simulink model "NonLinearModel"  (R2023b)
settings: Solver=ode45  StartTime=0.0  StopTime=Tsim*1.4  RelTol=1e-10  EnableMultiTasking=on
values from neighbouring files (symbols this model uses):
  alpha_init = 1*x_trim(1)    [FLYmodel.m]
  b = 9.17    [MyAircraft.mat]    (also in longMotion.m = 2.15; trimConfig.m)
  c = 2.15    [MyAircraft.mat]    (also in trimConfig.m)
  CG = 0.245    [MyAircraft.mat]    (also in trimConfig.m)
  el_init = x_trim(2)    [FLYmodel.m]
  eng_init = x_trim(4)    [FLYmodel.m]
  H_init = plane.h    [FLYmodel.m]
  Jgross = [5000 34000 45000 2200]    [MyAircraft.mat]    (also in trimConfig.m = [Ixx Iyy Izz Ixz])
  longK = lqr(podelny_system,Q,R)    [LQnavrh.m]
  m = 6500    [MyAircraft.mat]    (also in input_param.m = str2double(answerX{3}); trimConfig.m = plane.m)
  pitch_init = 1*x_trim(3)    [FLYmodel.m]
  plane = input_param    [FLYmodel.m]    (also in MyAircraft.mat = )
  rAC = 0.245    [MyAircraft.mat]    (also in trimConfig.m = plane.x_T)
  rho = 0.320310691736    [MyAircraft.mat]    (also in input_param.m = rho_0*(1-vyska/44308)^4.2553; trimConfig.m = plane.rho)
  S = 18.8    [MyAircraft.mat]    (also in latMotion.m; longMotion.m; trimConfig.m)
  Ts = 1/50    (= 0.02)    [FLYmodel.m]
  v0 = plane.v0    [FLYmodel.m]    (also in MyAircraft.mat = 187; input_param.m = str2double(answerX{1}); trimConfig.m)
  V_init = [plane.v0*cos(x_trim(1)) 0 plane.v0*sin(x_trim(1))]'    [FLYmodel.m]
  x_trim = trimConfig(plane)    [FLYmodel.m]    (also in MyAircraft.mat = [0.106204510792 -0.023384072427 0.106204510792 11783.3986038; trimConfig.m = [x(1) x(2) x(3) x(4)])
undefined symbols (not defined in the file or in its folder): Ap, As, Bp, Bs, Cp, Cs, Dp, Ds
libraries: simulink_extras x18
(part 1 of 2)
settings Model: Creator=Beruska  LastModifiedBy=cigla
settings SolverCC: ZeroCrossAlgorithm=Non-adaptive  AlgebraicLoopSolver=TrustRegion
settings DataIOCC: LimitDataPoints=on  SaveFormat=Array  SignalLoggingSaveFormat=ModelDataLogs  ReturnWorkspaceOutputs=off
settings OptimizationCC: ExpressionDepthLimit=2147483647  InitFltsAndDblsToZero=on  LifeSpan=inf
settings DebuggingCC: SaveWithDisabledLinksMsg=none  SaveWithParameterizedLinksMsg=none  UnderspecifiedInitializationDetection=Classic  MergeDetectMultiDrivingBlocksExec=none  SignalResolutionControl=TryResolveAllWithWarning  MultiTaskDSMMsg=warning  MultiTaskCondExecSysMsg=none  FcnCallInpInsideContextMsg=warning  StateNameClashWarn=warning  SFUnexpectedBacktrackingDiag=warning  SFNoUnconditionalDefaultTransitionDiag=warning  SFExecutionAtInitializationDiag=none  ArithmeticOperatorsInVariantConditions=warning
settings HardwareCC: ProdBitPerPointer=32  ProdBitPerSizeT=32  ProdBitPerPtrDiffT=32  ProdLargestAtomicFloat=None  ProdIntDivRoundTo=Undefined  ProdEndianess=Unspecified  ProdWordSize=32  ProdHWDeviceType=32-bit Generic  TargetHWDeviceType=32-bit Generic
settings ModelReferenceCC: PropagateSignalLabelsOutOfModel=off
settings SFSimCC: SimParseCustomCode=off
settings CodeAppCC: StateflowObjectComments=on
settings GRTTargetCC: TargetFcnLib=ansi_tfl_tmw.mat  TargetLangStandard=C89/C90 (ANSI)  CombineOutputUpdateFcns=off  GRTInterface=on
settings ConfigComp: CovMetricSettings=dw  CovSaveCumulativeToWorkspaceVar=on  CovSaveSingleToWorkspaceVar=on

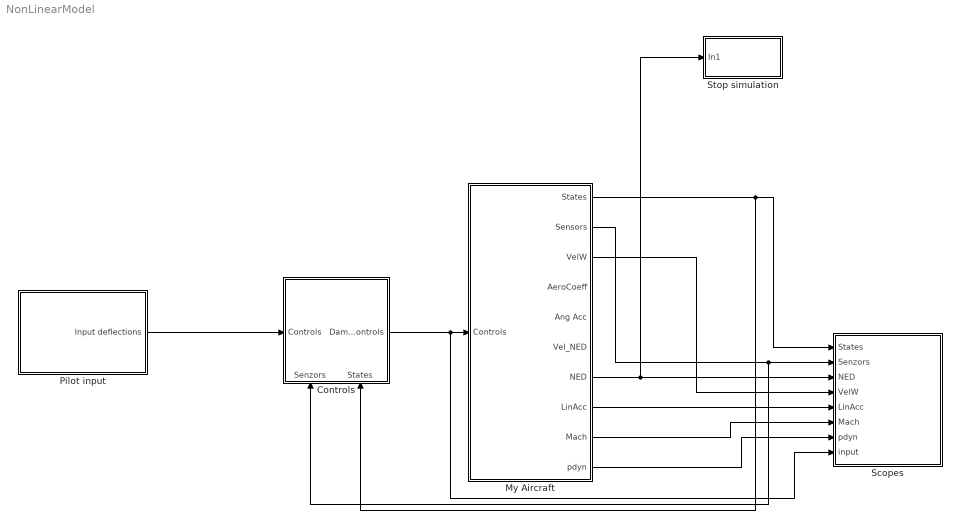
== system NonLinearModel ==
  Controls : Subsystem
      settings: PortSchema="{\"entries\":[{\"content\":{\"sides\":[{\"content\":{\"connectorIds\":[\"In1\"]},\"type\":\"ConnectorPlacement.EquallySpacedRectSide\",\"uuid\":\"4b7104ba-33e9-4b34-bfe8-b4b6035b4af3\"},{\"content\":{\"connectorIds\":[\"Out1\"],\"side\":\"RIGHT\"},\"type\":\"ConnectorPlacement.EquallySpacedRectSide\",\"uuid\":\"7145cc92-5786-41d0-90fc-f90dc0f3b476\"},{\"content\":{\"side\":\"TOP\"},\"type\":\"ConnectorPlacement.EquallySpacedRectSide\",\"uuid\":\"eba59bfa-479c-4b8a-8384-c15642ccc9eb\"},{\"content\":{\"connectorIds\":[\"In2\",\"In3\"],\"side\":\"BOTTOM\"},\"type\":\"ConnectorPlacement.EquallySpacedRectSide\",\"uuid\":\"538b7866-be33-4433-b066-8ee0a3ce190d\"}]},\"type\":\"ConnectorPlacement.EquallySpacedConnector\",\"uuid\":\"caacbf69-b2ca-40be-96e6-630faa4c76a7\"}],\"packageUris\":[\"http://schema.mathworks.com/mf0/Connector/R2020b\"],\"version\":\"1.0\"}"
  My Aircraft : Subsystem  mask(6-DOF Aircraft Model){aircraftcfg='MyAircraft.mat', VelocitiesIni=V_init, RatesIni=[0 0 0]', EulerIni=[0 pitch_init 0], PositionIni=[45/180*pi 45/180*pi H_init], QuatIni=[1 0 0 0], tsamp=Ts}
      mask prompts: aircraftcfg "Aircraft configuration file:"; VelocitiesIni "Initial velocities:"; RatesIni "Initial angular rates:"; EulerIni "Initial Euler:"; PositionIni "Initial position:"; QuatIni "Initial attitude:"; tsamp "Sample time:"
      mask help: Nonlinear 6-DOF aircraft model with equations of motion in body frame.
      mask init:
      | load(aircraftcfg);
      mask Help:
      | The block implements the 6-DOF nonlinear aircraft model using AeroSim blocks. Velocities are computed in body frame.
      | <P><B>Inputs:</B>
      | <LI>Controls = the 7x1 vector of aircraft controls [flap elevator aileron rudder throttle mixture ignition]. Aerodynamic controls are in radians, throttle is from 0 to 1, mixture is fraction air/fuel flow, ignition is 0 (engine off) or 1 (engine on).</LI>
      | <LI>Winds = the 3x1 vector of background wind speed components in navigation frame [North East Down]</LI>
      | <LI>RST = the integrator reset flag (0 or 1, all integrators on rising edge)
      | </P>
      | <P><B>Outputs:</B>
      | <LI>States = the 15x1 aircraft state vector [Velocities, Angular rates, Quaternions, Position, Fuel mass, Engine speed].</LI>
      | <LI>Sensors = the 18x1 vector of sensor outputs [GPS Position, GPS Groundspeed, Accelerometers, Gyros, Air data, Magnetometer].</LI>
      | <LI>VelW = the 3x1 vector of aircraft velocity in wind axes [Airspeed, sideslip, angle of attack]</LI>
      | <LI>Mach = the Mach number</LI>
      | <LI>Ang Acc = the 3x1 vector of angular accelerations
      | <LI>Euler = the 3x1 vector of Euler angles (roll, pitch, yaw)</LI>
      | <LI>AeroCoeff = the 6x1 vector of aerodynamic coefficients [CD CY CL Cl Cm Cn]</LI>
      | <LI>PropCoeff = the 3x1 vector of propeller coefficients [J CT CP]</LI>
      | <LI>EngCoeff = the 5x1 vector of engine coefficients [MAP Airflow Fuelflow BSFC Power]</LI>
      | <LI>Mass = the current aircraft mass</LI>
      | <LI>ECEF = 3x1 vector of position of the aircraft in the Earth-centered, Earth-fixed frame</LI>
      | <LI>MSL = the aircraft altitude above mean-sea-level</LI>
      | <LI>AGL = the aircraft altitude above terrain</LI>
      | <LI>REarth = the Earth equivalent radius at current location
      | <LI>AConGnd = the aircraft-on-ground flag (0 if aircraft above ground, 1 if aircraft on the ground)</LI>
      | </P>
      | <P><B>Parameters:</B>
      | <LI>Aircraft configuration file = the MAT-file with aircraft data</LI>
      | <LI>Initial velocities = the 3x1 vector of initial aircraft velocities in body axes [u v w]</LI>
      | <LI>Initial angular rates = the 3x1 vector of initial angular rates [p q r]</LI>
      | <LI>Initial attitude = the 4x1 vector of initial quaternions [e0 ex ey ez]</LI>
      | <LI>Initial position = the 3x1 vector of initial aircraft location [Lat Lon Alt]</LI>
      | <LI>Initial fuel mass = the initial quantity of fuel on-board the aircraft</LI>
      | <LI>Initial engine speed = the initial engine rotation speed</LI>
      | <LI>Ground altitude = the ground altitude at aircraft location</LI>
      | <LI>WMM coefficient file = the path to the magnetic model coefficient file</LI>
      | <LI>Simulation date = the date to be used for the magnetic model [day month year]</LI>
      | <LI>Sample time = the aircraft model sample time.</LI>
      | </P>
  Pilot input : Subsystem
  Scopes : Subsystem
  Stop simulation : Subsystem
  wires:
  My Aircraft/3(VelW) -> Scopes/4(VelW)
  My Aircraft/2(Sensors) -> Scopes/2(Senzors), Controls/2(Senzors)
  My Aircraft/7(NED) -> Stop simulation/1(In1), Scopes/3(NED)
  My Aircraft/1(States) -> Scopes/1(States), Controls/3(States)
  My Aircraft/8(LinAcc) -> Scopes/5(LinAcc)
  My Aircraft/9("Mach ") -> Scopes/6(Mach)
  My Aircraft/10(pdyn) -> Scopes/7(pdyn)
  Pilot input/1(Input deflections) -> Controls/1(Controls)
  Controls/1(Damped controls) -> Scopes/8(input), My Aircraft/1(Controls)

== system NonLinearModel/Controls ==
  Controls : Inport
  Senzors : Inport  Port=2
  States : Inport  Port=3
  Add1 : Sum
  Damping of controls : Subsystem
  Delay : Delay  DelayLength=10
  Knob : KnobBlock  ScaleMin=-90  ScaleMax=90
  Knob1 : KnobBlock  ScaleMin=-90  ScaleMax=90
  Manual Switch : ManualSwitch
  Subsystem : Subsystem
  Subsystem1 : Subsystem
  pitch : Constant  Value=8.570086669921878
  roll : Constant  Value=0  OutDataTypeStr=Inherit: Inherit via back propagation
  Damped controls : Outport
  wires:
  Senzors/1 -> Subsystem1/1(In1), Damping of controls/2(Senzors), Subsystem/3(sensors)
  Controls/1 -> Add1/1
  Damping of controls/1(Damped controls) -> Damped controls/1  "Damped controls"
  Add1/1 -> Damping of controls/1(Controls from pilot)
  roll/1 -> Delay/1  "roll"
  pitch/1 -> Subsystem/2(pitch setpoint)
  Manual Switch/1 -> Add1/2
  Delay/1 -> Subsystem/1(roll stepoint)
  States/1 -> Subsystem/4(States)
  Subsystem/1(Out1) -> Manual Switch/1

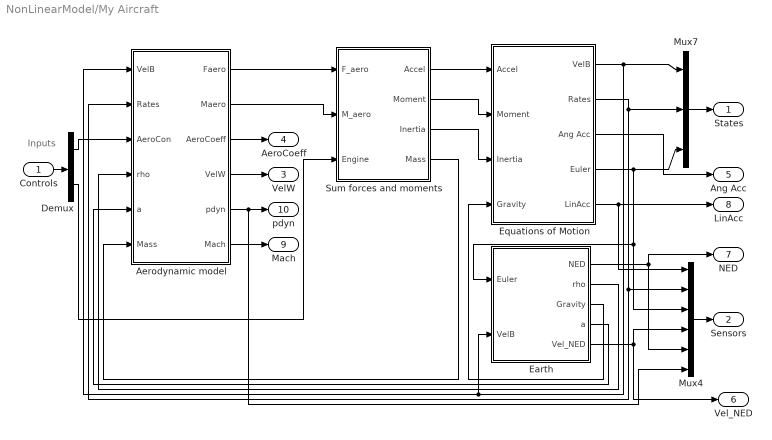
== system NonLinearModel/My Aircraft ==
  note: Inputs
  Controls : Inport
  Aerodynamic model : Subsystem
  Demux : Demux  Outputs=[3 1]
      settings: DisplayOption=none
  Earth : Subsystem
  Equations of Motion : Subsystem
  Mux4 : Mux  Inputs=6
  Mux7 : Mux  Inputs=3
  Sum forces and moments : Subsystem
  States : Outport
  Sensors : Outport  Port=2
  VelW : Outport  Port=3
  AeroCoeff : Outport  Port=4
  Ang Acc : Outport  Port=5
  Vel_NED : Outport  Port=6
  NED : Outport  Port=7
  LinAcc : Outport  Port=8
  "Mach " : Outport  Port=9
  pdyn : Outport  Port=10
  wires:
  Controls/1 -> Demux/1
  Mux4/1 -> Sensors/1
  Mux7/1 -> States/1
  Equations of Motion/1(VelB) -> Mux7/1, Aerodynamic model/1(VelB), Earth/2(VelB)
  Equations of Motion/2(Rates) -> Aerodynamic model/2(Rates), Mux4/2, Mux7/2
  Aerodynamic model/3(AeroCoeff) -> AeroCoeff/1
  Demux/1 -> Aerodynamic model/3(AeroCon)
  Earth/3(Gravity) -> Equations of Motion/4(Gravity)
  Equations of Motion/4(Euler) -> Mux7/3, Mux4/3, Earth/1(Euler)
  Aerodynamic model/1(Faero) -> Sum forces and moments/1(F_aero)
  Aerodynamic model/2(Maero) -> Sum forces and moments/2(M_aero)
  Demux/2 -> Sum forces and moments/3(Engine)
  Sum forces and moments/1(Accel) -> Equations of Motion/1(Accel)
  Sum forces and moments/2(Moment) -> Equations of Motion/2(Moment)
  Sum forces and moments/3(Inertia) -> Equations of Motion/3(Inertia)
  Earth/4(a) -> Aerodynamic model/5(a)
  Earth/2(rho) -> Aerodynamic model/4(rho)
  Earth/1(NED) -> Mux4/5, NED/1
  Aerodynamic model/5(pdyn) -> Mux4/6, pdyn/1
  Sum forces and moments/4(Mass) -> Aerodynamic model/6(Mass)
  Equations of Motion/3(Ang Acc) -> Ang Acc/1
  Equations of Motion/5(LinAcc) -> LinAcc/1, Mux4/1
  Aerodynamic model/6("Mach ") -> "Mach "/1
  Earth/5(Vel_NED) -> Vel_NED/1, Mux4/4
  Aerodynamic model/4(VelW) -> VelW/1

== system NonLinearModel/Pilot input ==
  Ground : Ground
  Ground1 : Ground
  Ground2 : Ground
  Manual Switch : ManualSwitch  CurrentSetting=0
  Manual Switch1 : ManualSwitch  CurrentSetting=0
  Manual Switch2 : ManualSwitch
  Mux3 : Mux
  Sum2 : Sum  Inputs=++|
  aileron : Subsystem
  elevator : Constant  Value=el_init
  elvator : Subsystem
  engine : Constant  Value=eng_init
  rudder : Subsystem
  Input deflections : Outport
  wires:
  engine/1 -> Mux3/4
  elevator/1 -> Sum2/2
  Sum2/1 -> Mux3/1
  Manual Switch/1 -> Mux3/2
  Ground/1 -> Manual Switch/2
  rudder/1(Out1) -> Manual Switch1/1  "rudder"
  Ground1/1 -> Manual Switch1/2
  Manual Switch1/1 -> Mux3/3
  elvator/1(Out1) -> Manual Switch2/1
  aileron/1(Out1) -> Manual Switch/1  "aileron"
  Ground2/1 -> Manual Switch2/2
  Manual Switch2/1 -> Sum2/1
  Mux3/1 -> Input deflections/1

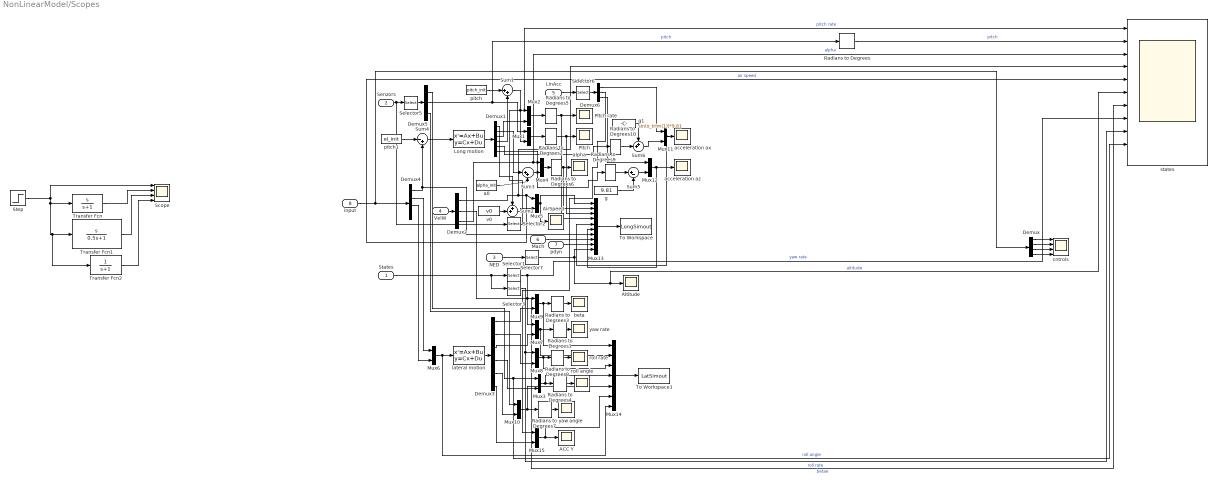
== system NonLinearModel/Scopes ==
  States : Inport
  Senzors : Inport  Port=2
  NED : Inport  Port=3
  VelW : Inport  Port=4
  LinAcc : Inport  Port=5
  Mach : Inport  Port=6
  pdyn : Inport  Port=7
  input : Inport  Port=8
  ACC Y : Scope
  AirSpeed : Scope
  Altitude : Scope
  Demux : Demux
  Demux1 : Demux  Outputs=6
      settings: DisplayOption=none
  Demux2 : Demux  Outputs=3
      settings: DisplayOption=none
  Demux3 : Demux  Outputs=6
      settings: DisplayOption=none
  Demux4 : Demux
      settings: DisplayOption=none
  Demux5 : Demux  Outputs=3
      settings: DisplayOption=none
  Demux6 : Demux  Outputs=3
      settings: DisplayOption=none
  Long motion : StateSpace  A=Ap  B=Bp  C=Cp  D=Dp  InitialCondition=0
  Mux{1..12,15} (13 alike) : Mux  Inputs=2
  Mux13 : Mux  Inputs=10
  Mux14 : Mux  Inputs=7
  Pitch : Scope
  Pitch rate : Scope
  Radians to Degrees{,1..8} (9 alike) : simulink_extras/Transformations/Radians to Degrees
  Radians to Degrees10 : simulink_extras/Transformations/Radians to Degrees
      link override Gain: Gain=9.81
  Radians to Degrees9 : simulink_extras/Transformations/Radians to Degrees
      link override Gain: Gain=-9.81
  Scope : Scope  NumInputPorts=4
  Selector1 : Selector  InputPortWidth=9  IndexOptions=Index vector (dialog)  Indices=6  OutputSizes=[(-2)]
  Selector2 : Selector  InputPortWidth=16  IndexOptions=Index vector (dialog)  Indices=5  OutputSizes=[(-2)]
  Selector3 : Selector  InputPortWidth=9  IndexOptions=Index vector (dialog)  Indices=4  OutputSizes=[(-2)]
  Selector5 : Selector  InputPortWidth=16  IndexOptions=Index vector (dialog)  Indices=[7 8 9]  OutputSizes=1
  Selector6 : Selector  InputPortWidth=3  IndexOptions=Index vector (dialog)  Indices=[1 2 3]  OutputSizes=1
  Selector7 : Selector  InputPortWidth=3  IndexOptions=Index vector (dialog)  Indices=3  OutputSizes=[(-2)]
  Step : Step  SampleTime=0
  Sum1 : Sum  Inputs=|++
  Sum2 : Sum  Inputs=++|
  Sum3 : Sum  Inputs=|++
  Sum4 : Sum  Inputs=|-+
  Sum5 : Sum  Inputs=|+-
  Sum6 : Sum  Inputs=++|
  To Workspace : ToWorkspace  VariableName=LongSimout  SaveFormat=Structure With Time  SampleTime=Ts
  To Workspace1 : ToWorkspace  VariableName=LatSimout  SaveFormat=Structure With Time  SampleTime=Ts
  Transfer Fcn : TransferFcn  Numerator=[1 0]  Denominator=[1 1]
  Transfer Fcn1 : TransferFcn  Numerator=[1 0]  Denominator=[0.5 1]
  Transfer Fcn2 : TransferFcn  Denominator=[1 1]
  a0 : Constant  Value=alpha_init
  acceleration ax : Scope
  acceleration az : Scope
  "alpha " : Scope
  beta : Scope
  cntrols : Scope  NumInputPorts=4
  g : Constant  Value=9.81
  g1 : Constant  Value=sin(x_trim(1))*9.81
  lateral motion : StateSpace  A=As  B=Bs  C=Cs  D=Ds  InitialCondition=0
  pitch : Constant  Value=pitch_init
  pitch1 : Constant  Value=el_init
  roll angle : Scope
  roll rate : Scope
  states : Scope  NumInputPorts=11
  v0 : Constant  Value=v0
  yaw angle : Scope
  yaw rate : Scope
  wires:
  Long motion/1 -> Demux1/1
  Demux1/4 -> Sum1/2
  Mux1/1 -> Radians to Degrees2/1
  pitch/1 -> Sum1/1
  Demux5/2 -> Radians to Degrees/1, Mux1/1  "pitch"
  Mux2/1 -> Radians to Degrees5/1
  Demux1/3 -> Mux2/2
  Mux4/1 -> Radians to Degrees6/1
  Demux1/2 -> Sum3/1
  Demux1/1 -> Sum2/1
  Mux5/1 -> AirSpeed/1, Mux13/1
  Sum2/1 -> Mux5/2
  v0/1 -> Sum2/2
  Sum3/1 -> Mux4/2
  a0/1 -> Sum3/2
  Selector1/1 -> Mux7/1, states/8  "yaw rate"
  Mux7/1 -> Mux14/2, Radians to Degrees1/1
  Radians to Degrees1/1 -> yaw rate/1
  Mux8/1 -> Radians to Degrees8/1, Mux14/3
  Radians to Degrees8/1 -> roll rate/1
  Selector3/1 -> Mux8/1, states/9  "roll rate"
  lateral motion/1 -> Demux3/1
  Mux9/1 -> Radians to Degrees3/1, Mux14/1
  Radians to Degrees3/1 -> beta/1
  Mux6/1 -> lateral motion/1, Mux14/7
  Demux4/3 -> Mux6/2
  Demux4/1 -> Sum4/2, Mux13/7
  Demux2/3 -> states/3, Mux4/1  "alpha"
  input/1 -> Demux/1, Demux4/1
  Demux4/2 -> Mux6/1
  Sum4/1 -> Long motion/1
  pitch1/1 -> Sum4/1
  Demux3/2 -> Mux8/2
  Demux3/1 -> Mux9/2
  VelW/1 -> Demux2/1
  Demux2/2 -> states/7, Mux9/1  "betae"
  Radians to Degrees6/1 -> "alpha "/1, Mux13/2
  Selector2/1 -> states/1, Mux2/1  "pitch rate"
  Radians to Degrees5/1 -> Pitch rate/1, Mux13/4
  Demux3/3 -> Mux7/2
  Mux3/1 -> Radians to Degrees4/1, Mux14/4
  Radians to Degrees4/1 -> roll angle/1
  Demux3/4 -> Mux3/2
  Senzors/1 -> Selector2/1, Selector5/1
  Demux5/3 -> Mux10/1
  Mux10/1 -> Radians to Degrees7/1, Mux14/5
  Radians to Degrees7/1 -> yaw angle/1
  Demux3/5 -> Mux10/2
  Demux5/1 -> Mux3/1, states/10  "roll angle"
  Selector5/1 -> Demux5/1
  Radians to Degrees2/1 -> Pitch/1, Mux13/3
  Sum1/1 -> Mux1/2
  States/1 -> Selector1/1, Selector3/1
  Demux2/1 -> states/5, Mux5/1, states/4  "air speed"
  Demux1/5 -> Radians to Degrees10/1
  Mux11/1 -> acceleration ax/1, Mux13/5
  Selector6/1 -> Demux6/1
  Demux6/1 -> Mux11/1
  Mux12/1 -> Mux13/6, acceleration az/1
  Demux6/3 -> Mux12/1
  Demux1/6 -> Radians to Degrees9/1
  Radians to Degrees9/1 -> Sum5/1
  LinAcc/1 -> Selector6/1
  g/1 -> Sum5/2
  Sum5/1 -> Mux12/2
  g1/1 -> Sum6/1
  Radians to Degrees10/1 -> Sum6/2
  Sum6/1 -> Mux11/2
  Mux13/1 -> To Workspace/1
  Mach/1 -> Mux13/8
  pdyn/1 -> Mux13/9
  NED/1 -> Selector7/1
  Selector7/1 -> Mux13/10, states/6, Altitude/1  "altitude"
  Mux14/1 -> To Workspace1/1
  Demux6/2 -> Mux15/1
  Mux15/1 -> ACC Y/1, Mux14/6
  Demux3/6 -> Mux15/2
  Transfer Fcn/1 -> Scope/2
  Step/1 -> Transfer Fcn/1, Transfer Fcn2/1, Transfer Fcn1/1, Scope/1
  Transfer Fcn1/1 -> Scope/3
  Transfer Fcn2/1 -> Scope/4
  Demux/1 -> cntrols/1
  Demux/2 -> cntrols/2
  Demux/3 -> cntrols/3
  Demux/4 -> cntrols/4
  Radians to Degrees/1 -> states/2  "pitch"

== system NonLinearModel/Stop simulation ==
  In1 : Inport
  Constant : Constant  Value=0
  Constant1 : Constant
  Demux : Demux  Outputs=[2 1]
  Scope1 : Scope
  Stop Simulation : Stop
  Switch : Switch  SaturateOnIntegerOverflow=off  InputSameDT=off
  Terminator : Terminator
  wires:
  Constant/1 -> Switch/1
  Constant1/1 -> Switch/3
  In1/1 -> Demux/1
  Demux/2 -> Switch/2
  Demux/1 -> Terminator/1
  Switch/1 -> Stop Simulation/1, Scope1/1

== system NonLinearModel/Controls/Damping of controls ==
  Controls from pilot : Inport
  Senzors : Inport  Port=2
  Add{,2..3,5} (4 alike) : Sum
  Demux1 : Demux  Outputs=3
  Demux2 : Demux
  Gain2 : Gain  Gain=0.07
  Ground : Ground
  Mux : Mux
  Subsystem : Subsystem
  Transfer Fcn : TransferFcn  Numerator=[1 0]  Denominator=[1 1]
  pitch damper : Gain  Gain=0.063
  roll damper : Gain  Gain=-0.054
  Damped controls : Outport
  wires:
  pitch damper/1 -> Add/2
  Add/1 -> Mux/1  "damped elevator"
  Demux2/1 -> Add/1  "elevator from pilot"
  Demux1/3 -> roll damper/1  "roll rate"
  Demux2/4 -> Add3/1  "Engine thrust from pilot"
  Demux2/3 -> Add5/1  "Rudder from pilot"
  Demux1/2 -> pitch damper/1  "pitch rate"
  Demux1/1 -> Gain2/1  "yaw rate"
  Add3/1 -> Mux/4  "engine"
  Add5/1 -> Mux/3  "damped rudder"
  Demux2/2 -> Add2/1  "Aileron from pilot"
  Add2/1 -> Mux/2  "damped ailerons"
  Controls from pilot/1 -> Demux2/1
  Mux/1 -> Damped controls/1
  roll damper/1 -> Add2/2
  Transfer Fcn/1 -> Add5/2
  Gain2/1 -> Transfer Fcn/1
  Ground/1 -> Add3/2
  Senzors/1 -> Subsystem/1(In1)
  Subsystem/1(Rates) -> Demux1/1

== system NonLinearModel/Controls/Subsystem ==
  roll stepoint : Inport
  pitch setpoint : Inport  Port=2
  sensors : Inport  Port=3
  States : Inport  Port=4
  Constant : Constant  Value=0
  Manual Switch : ManualSwitch  CurrentSetting=0
  Mux : Mux
  PAH : Subsystem
  PAH_LQ : Subsystem
  RAH : Subsystem
  RAH_LQ : Subsystem
  demuxing hell : Subsystem
  Out1 : Outport
  wires:
  Mux/1 -> Out1/1
  roll stepoint/1 -> RAH/1(In1)
  RAH/1(Out1) -> Mux/2  "aileron"
  pitch setpoint/1 -> PAH_LQ/1(pitch setpoint), PAH/1(pitch setpoint)
  Manual Switch/1 -> Mux/1  "elevator"
  ? -> Mux/3  "rudder"
  ? -> Mux/4  "engine"
  sensors/1 -> demuxing hell/1(sensors)
  States/1 -> demuxing hell/2(In2)
  demuxing hell/1(pitch) -> PAH/2(pitch)
  demuxing hell/2(roll) -> RAH/2(roll)
  demuxing hell/3(long states) -> PAH_LQ/2(long states)
  PAH/1(Out1) -> Manual Switch/1  "elevator"
  PAH_LQ/1(Out1) -> Manual Switch/2

== system NonLinearModel/Controls/Subsystem1 ==
  In1 : Inport
  Demux : Demux  Outputs=6
  Terminator{,1..5} (6 alike) : Terminator
  wires:
  Demux/1 -> Terminator/1  "Lin Acc"
  Demux/2 -> Terminator1/1  "Rates"
  Demux/3 -> Terminator5/1  "Euler Angles"
  Demux/5 -> Terminator3/1  "NED"
  Demux/4 -> Terminator2/1  "Velocity NED"
  Demux/6 -> Terminator4/1  "dynamic pressure"
  In1/1 -> Demux/1

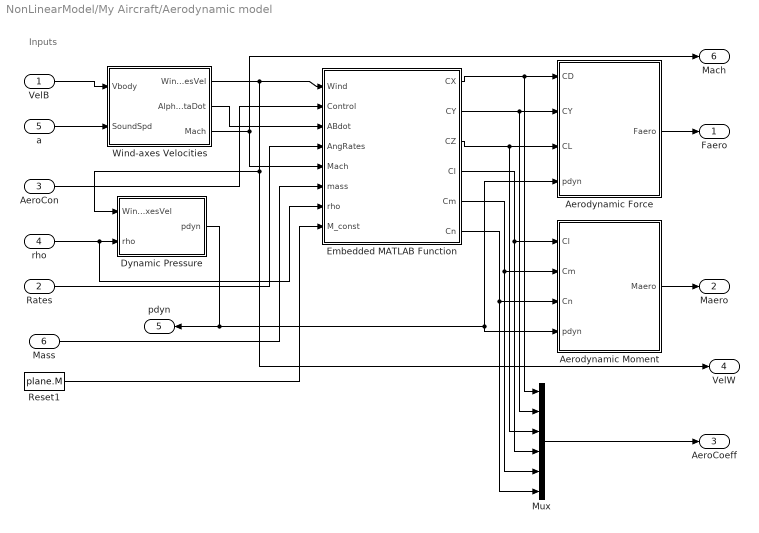
== system NonLinearModel/My Aircraft/Aerodynamic model ==
  note: Inputs
  VelB : Inport  PortDimensions=[3 1]
  Rates : Inport  Port=2  PortDimensions=[3 1]
  AeroCon : Inport  Port=3
  rho : Inport  Port=4  PortDimensions=1
  a : Inport  Port=5  PortDimensions=1
  Mass : Inport  Port=6
  Aerodynamic Force : Subsystem  mask(Aerodynamic force){S=S}
      mask prompts: S "Wing reference area:"
      mask help: Computes aerodynamic force in body axes.
      mask Help:
      | The block computes the aerodynamic force in body axes.
      | <P><B>Inputs:</B>
      | <LI>CD = the coefficient of drag</LI>
      | <LI>CY = the coefficient of side force</LI>
      | <LI>CL = the coefficient of lift</LI>
      | <LI>pdyn = the dynamic pressure</LI>
      | <LI>WindAxesVel = the 3x1 vector of wind axes velocity components [Va beta alpha]'</LI>
      | </P>
      | <P><B>Output:</B> the 3x1 vector of aerodynamic forces in body axes</P>
      | <P><B>Parameters:</B>
      | <LI>S = the wing reference area</LI>
      | </P>
  Aerodynamic Moment : Subsystem  mask(Aerodynamic moment){c=c, b=b, S=S}
      mask prompts: c "Mean aerodynamic chord:"; b "Wing span:"; S "Wing reference area:"
      mask help: Computes aerodynamic moment with respect to the aerodynamic center.
  Dynamic Pressure : Subsystem
  Embedded MATLAB Function : MATLAB Function  TreatAsAtomicUnit=on
  Mux : Mux  Inputs=6
  Reset1 : Constant  Value=plane.M
  Wind-axes Velocities : Subsystem
  Faero : Outport
  Maero : Outport  Port=2
  AeroCoeff : Outport  Port=3
  VelW : Outport  Port=4
  pdyn : Outport  Port=5
  "Mach " : Outport  Port=6
  wires:
  Rates/1 -> Embedded MATLAB Function/4(AngRates)
  Aerodynamic Moment/1(Maero) -> Maero/1
  Aerodynamic Force/1(Faero) -> Faero/1
  Dynamic Pressure/1(pdyn) -> Aerodynamic Moment/4(pdyn), Aerodynamic Force/4(pdyn), pdyn/1
  Wind-axes Velocities/2(AlphaBetaDot) -> Embedded MATLAB Function/3(ABdot)
  rho/1 -> Dynamic Pressure/2(rho), Embedded MATLAB Function/7(rho)
  Wind-axes Velocities/1(WindAxesVel) -> Dynamic Pressure/1(WindAxesVel), VelW/1, Embedded MATLAB Function/1(Wind)
  a/1 -> Wind-axes Velocities/2(SoundSpd)
  VelB/1 -> Wind-axes Velocities/1(Vbody)
  Wind-axes Velocities/3(Mach) -> "Mach "/1, Embedded MATLAB Function/5(Mach)
  AeroCon/1 -> Embedded MATLAB Function/2(Control)
  Embedded MATLAB Function/1(CX) -> Aerodynamic Force/1(CD), Mux/1
  Embedded MATLAB Function/3(CZ) -> Aerodynamic Force/3(CL), Mux/3
  Embedded MATLAB Function/5(Cm) -> Aerodynamic Moment/2(Cm), Mux/5
  Embedded MATLAB Function/2(CY) -> Aerodynamic Force/2(CY), Mux/2
  Embedded MATLAB Function/6(Cn) -> Aerodynamic Moment/3(Cn), Mux/6
  Reset1/1 -> Embedded MATLAB Function/8(M_const)
  Embedded MATLAB Function/4(Cl) -> Aerodynamic Moment/1(Cl), Mux/4
  Mass/1 -> Embedded MATLAB Function/6(mass)
  Mux/1 -> AeroCoeff/1

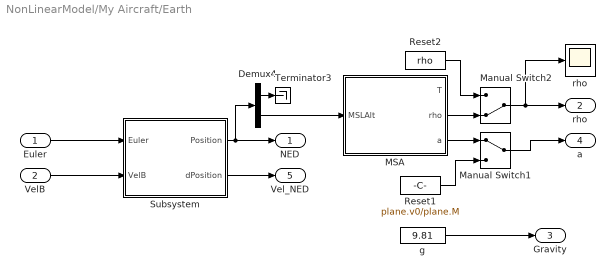
== system NonLinearModel/My Aircraft/Earth ==
  Euler : Inport  OutDataTypeStr=double
  VelB : Inport  Port=2  OutDataTypeStr=double
  Demux4 : Demux  Outputs=[2 1]
      settings: DisplayOption=none
  MSA : Subsystem
  Manual Switch1 : ManualSwitch
  Manual Switch2 : ManualSwitch  CurrentSetting=0
  Reset1 : Constant  Value=plane.v0/plane.M
  Reset2 : Constant  Value=rho
  Subsystem : Subsystem
  Terminator3 : Terminator
  g : Constant  Value=9.81
  "rho " : Scope
  NED : Outport
  rho : Outport  Port=2
  Gravity : Outport  Port=3
  a : Outport  Port=4
  Vel_NED : Outport  Port=5
  wires:
  g/1 -> Gravity/1
  MSA/3(a) -> Manual Switch1/1
  Manual Switch1/1 -> a/1
  MSA/2(rho) -> Manual Switch2/2
  Reset2/1 -> Manual Switch2/1
  Manual Switch2/1 -> rho/1, "rho "/1
  Demux4/1 -> Terminator3/1
  Subsystem/1(Position) -> Demux4/1, NED/1
  Reset1/1 -> Manual Switch1/2
  Euler/1 -> Subsystem/1(Euler)
  VelB/1 -> Subsystem/2(VelB)
  Demux4/2 -> MSA/1(MSLAlt)
  Subsystem/2(dPosition) -> Vel_NED/1

== system NonLinearModel/My Aircraft/Equations of Motion ==
  note: Inputs
  note: Outputs
  Accel : Inport  PortDimensions=[3 1]
  Moment : Inport  Port=2  PortDimensions=[3 1]
  Inertia : Inport  Port=3  PortDimensions=[4 1]
  Gravity : Inport  Port=4
  Forces : Subsystem  mask(Force equations){VelocitiesIni=VelocitiesIni}
      mask prompts: VelocitiesIni "Initial velocities:"
      mask help: 6-DOF rigid body force equations.
      mask Help:
      | The block implements the 6-DOF rigid-body force equations.
      | <P><B>Inputs:</B>
      | <LI>Rates = the 3x1 vector of body angular rates</LI>
      | <LI>Accel = the 3x1 vector of linear body accelerations</LI>
      | <LI>Gravity = the gravitational acceleration at current location.
      | <LI>DCM = the 3x3 rotation matrix from navigation to body frame.
      | <LI>RST = the integrator reset flag (rising edge)</LI>
      | </P>
      | <P><B>Output:</B>
      | <LI>Velocities = the 3x1 vector of aircraft velocities in body axes</LI>
      | </P>
      | <P><B>Parameters:</B>
      | <LI>Initial velocities = the 3x1 vector of initial aircraft velocities</LI>
      | </P>
  Kinematics (Euler) : Subsystem  mask(Kinematic Equations){EulerIniX=EulerIni}
      mask prompts: EulerIniX "Initial Euler:"
      mask help: 6-DOF rigid body kinematic equations, using Euler-Rodrigues quaternions.
      mask Help:
      | The block implements the 6-DOF rigid-body kinematic equations, using Euler-Rodrigues quaternions.
      | <P><B>Inputs:</B>
      | <LI>Rates = the 3x1 vector of body angular rates</LI>
      | <LI>RST = the integrator reset flag (rising edge)</LI>
      | </P>
      | <P><B>Output:</B>
      | <LI>Quaternions = the 4x1 vector of body quaternions</LI>
      | </P>
      | <P><B>Parameters:</B>
      | <LI>Initial quaternions = the 4x1 vector of initial body quaternions</LI>
      | </P>
  Moments : Subsystem  mask(Moment equations){RatesIni=RatesIni}
      mask prompts: RatesIni "Initial angular rates:"
      mask help: 6-DOF rigid body moment equations.
      mask Help:
      | The block implements the 6-DOF rigid-body moment equations.
      | <P><B>Inputs:</B>
      | <LI>Inertia = the 10x1 vector of inertia coefficients</LI>
      | <LI>Moments = the 3x1 vector of airframe moments</LI>
      | <LI>RST = the integrator reset flag (rising edge)</LI>
      | </P>
      | <P><B>Output:</B>
      | <LI>Angular Rates = the 3x1 vector of body angular rates</LI>
      | <LI>Angular Acc = the 3x1 vector of body angular accelerations.
      | </P>
      | <P><B>Parameters:</B>
      | <LI>Initial rates = the 3x1 vector of initial angular rates</LI>
      | </P>
  VelB : Outport
  Rates : Outport  Port=2
  Ang Acc : Outport  Port=3
  Euler : Outport  Port=4
  LinAcc : Outport  Port=5
  wires:
  Moments/2(Angular Acc) -> Ang Acc/1
  Moments/1(Angular Rates) -> Rates/1, Kinematics (Euler)/1(Rates), Forces/1(Rates)
  Forces/1(Velocities) -> VelB/1
  Inertia/1 -> Moments/1(Inertia)
  Moment/1 -> Moments/2(Moments)
  Accel/1 -> Forces/2(Accel)
  Kinematics (Euler)/1(Euler) -> Forces/3(Euler), Euler/1
  Gravity/1 -> Forces/4(Gravity)
  Forces/2(LinAcc) -> LinAcc/1

== system NonLinearModel/My Aircraft/Sum forces and moments ==
  F_aero : Inport
  M_aero : Inport  Port=2
  Engine : Inport  Port=3
  CG location : Constant  Value=CG
  Mass gross : Constant  Value=m
  Moments of inertia : Constant  Value=Jgross
  Total Acceleration : Subsystem
  Total Moment : Subsystem
  Accel : Outport
  Moment : Outport  Port=2
  Inertia : Outport  Port=3
  Mass : Outport  Port=4
  wires:
  Mass gross/1 -> Total Acceleration/2(Mass), Mass/1
  CG location/1 -> Total Moment/3(CGpos)
  F_aero/1 -> Total Moment/1(Faero), Total Acceleration/1(Faero)
  Total Acceleration/1(Acc) -> Accel/1
  Engine/1 -> Total Acceleration/3(Engine)
  M_aero/1 -> Total Moment/2(Maero)
  Total Moment/1(Mcg) -> Moment/1
  Moments of inertia/1 -> Inertia/1

== system NonLinearModel/Pilot input/aileron ==
  Gain : Gain
  Manual Switch : ManualSwitch
  Radians to Degrees11 : simulink_extras/Transformations/Radians to Degrees
  Step : Step  Time=40  After=20/180*pi  SampleTime=0
  Step1 : Step  Time=50  After=-40/180*pi  SampleTime=0
  Step2 : Step  Time=60  After=20/180*pi  SampleTime=0
  Step3 : Step  Time=5  After=20/180*pi  SampleTime=0
  Sum4 : Sum  Inputs=3
  input : Scope
  phugoid : Gain  Gain=-1/10000
  short period : Gain  Gain=-1/100
  Out1 : Outport
  wires:
  Sum4/1 -> short period/1
  Step/1 -> Sum4/1
  Step1/1 -> Sum4/2
  Step2/1 -> Sum4/3
  Manual Switch/1 -> Radians to Degrees11/1, Out1/1
  Radians to Degrees11/1 -> input/1
  short period/1 -> Manual Switch/1
  Step3/1 -> phugoid/1
  phugoid/1 -> Gain/1
  Gain/1 -> Manual Switch/2

== system NonLinearModel/Pilot input/elvator ==
  Gain : Gain  Gain=1000
  Manual Switch : ManualSwitch  CurrentSetting=0
  Radians to Degrees11 : simulink_extras/Transformations/Radians to Degrees
  Step : Step  Time=5  After=20/180*pi  SampleTime=0
  Step1 : Step  Time=15  After=-40/180*pi  SampleTime=0
  Step2 : Step  Time=25  After=20/180*pi  SampleTime=0
  Step3 : Step  Time=5  After=20/180*pi  SampleTime=0
  Sum4 : Sum  Inputs=3
  input : Scope
  phugoid : Gain  Gain=-1/10000
  short period : Gain  Gain=-1/100
  Out1 : Outport
  wires:
  Sum4/1 -> short period/1
  Step/1 -> Sum4/1
  Step1/1 -> Sum4/2
  Step2/1 -> Sum4/3
  Manual Switch/1 -> Radians to Degrees11/1, Out1/1
  Radians to Degrees11/1 -> input/1
  short period/1 -> Manual Switch/1
  Step3/1 -> phugoid/1
  phugoid/1 -> Gain/1
  Gain/1 -> Manual Switch/2

== system NonLinearModel/Pilot input/rudder ==
  Gain : Gain  Gain=1000
  Manual Switch : ManualSwitch
  Radians to Degrees11 : simulink_extras/Transformations/Radians to Degrees
  Step : Step  Time=5  After=20/180*pi  SampleTime=0
  Step1 : Step  Time=15  After=-40/180*pi  SampleTime=0
  Step2 : Step  Time=25  After=20/180*pi  SampleTime=0
  Step3 : Step  Time=5  After=20/180*pi  SampleTime=0
  Sum4 : Sum  Inputs=3
  input : Scope
  phugoid : Gain  Gain=-1/10000
  short period : Gain  Gain=-1/100
  Out1 : Outport
  wires:
  Gain/1 -> Manual Switch/2
  phugoid/1 -> Gain/1
  Step3/1 -> phugoid/1
  short period/1 -> Manual Switch/1
  Radians to Degrees11/1 -> input/1
  Manual Switch/1 -> Out1/1, Radians to Degrees11/1
  Step2/1 -> Sum4/3
  Step1/1 -> Sum4/2
  Step/1 -> Sum4/1
  Sum4/1 -> short period/1

== system NonLinearModel/Controls/Damping of controls/Subsystem ==
  In1 : Inport
  Demux : Demux  Outputs=6
  Terminator{,1..4} (5 alike) : Terminator
  Rates : Outport
  wires:
  Demux/4 -> Terminator2/1  "Velocity NED"
  Demux/6 -> Terminator4/1  "dynamic pressure"
  Demux/1 -> Terminator/1  "Lin Acc"
  In1/1 -> Demux/1
  Demux/5 -> Terminator3/1  "NED"
  Demux/3 -> Terminator1/1  "Euler Angles"
  Demux/2 -> Rates/1  "Rates"

== system NonLinearModel/Controls/Subsystem/PAH ==
  pitch setpoint : Inport
  pitch : Inport  Port=2
  Add : Sum
  Gain : Gain  Gain=0.01
  Gain1 : Gain  Gain=-1
  Gain2 : Gain  Gain=0.01
  Integrator : Integrator
  Radians to Degrees : simulink_extras/Transformations/Radians to Degrees
  Subtract1 : Sum  Inputs=+-
  Out1 : Outport
  wires:
  Subtract1/1 -> Gain2/1, Gain/1  "pitch error"
  pitch setpoint/1 -> Subtract1/1
  pitch/1 -> Radians to Degrees/1
  Gain1/1 -> Out1/1
  Radians to Degrees/1 -> Subtract1/2
  Add/1 -> Gain1/1
  Gain/1 -> Add/1
  Integrator/1 -> Add/2
  Gain2/1 -> Integrator/1

== system NonLinearModel/Controls/Subsystem/PAH_LQ ==
  pitch setpoint : Inport
  long states : Inport  Port=2
  0 because LQR drives states to 0 : Constant  Value=0
  Degrees to Radians : simulink_extras/Transformations/Degrees to Radians
  Demux : Demux  Outputs=5
  Display : Display
  Gain : Gain  Gain=longK  Multiplication=Matrix(K*u)
  Gain1 : Gain
  Integrator : Integrator
  Mux : Mux
  Subsystem : Subsystem
  Subtract1 : Sum  Inputs=-+
  Out1 : Outport
  wires:
  Demux/4 -> Subtract1/1  "pitch"
  pitch setpoint/1 -> Degrees to Radians/1
  Gain1/1 -> Out1/1
  Gain/1 -> Gain1/1
  long states/1 -> Demux/1
  Demux/2 -> Mux/2  "angle of attack"
  Demux/3 -> Mux/3  "pitch rate"
  Degrees to Radians/1 -> Subtract1/2
  Mux/1 -> Gain/1, Subsystem/2(states)
  Subtract1/1 -> Integrator/1  "pitch error"
  Integrator/1 -> Mux/4, Display/1
  0 because LQR drives states to 0/1 -> Mux/1
  Demux/1 -> Subsystem/1(velocity)  "velocity"
  Demux/5 -> Subsystem/3(altitude)  "altitude"

== system NonLinearModel/Controls/Subsystem/RAH ==
  In1 : Inport
  roll : Inport  Port=2
  Add : Sum
  Gain : Gain  Gain=0.001
  Gain1 : Gain  Gain=-1
  Gain2 : Gain  Gain=0.00005
  Integrator : Integrator  LimitOutput=on  UpperSaturationLimit=0.01  LowerSaturationLimit=-0.01
  Radians to Degrees : simulink_extras/Transformations/Radians to Degrees
  Subtract : Sum  Inputs=+-
  Out1 : Outport
  wires:
  Subtract/1 -> Gain/1, Gain2/1  "roll error"
  Add/1 -> Gain1/1
  In1/1 -> Subtract/1
  roll/1 -> Radians to Degrees/1
  Radians to Degrees/1 -> Subtract/2
  Gain1/1 -> Out1/1
  Gain2/1 -> Integrator/1
  Integrator/1 -> Add/2
  Gain/1 -> Add/1

== system NonLinearModel/Controls/Subsystem/RAH_LQ ==
  In1 : Inport
  roll : Inport  Port=2
  Add : Sum
  Gain : Gain  Gain=0.001
  Gain1 : Gain  Gain=-1
  Gain2 : Gain  Gain=0.00005
  Integrator : Integrator  LimitOutput=on  UpperSaturationLimit=0.01  LowerSaturationLimit=-0.01
  Radians to Degrees : simulink_extras/Transformations/Radians to Degrees
  Subtract : Sum  Inputs=+-
  Out1 : Outport
  wires:
  Subtract/1 -> Gain/1, Gain2/1  "roll error"
  Add/1 -> Gain1/1
  In1/1 -> Subtract/1
  roll/1 -> Radians to Degrees/1
  Radians to Degrees/1 -> Subtract/2
  Gain1/1 -> Out1/1
  Gain2/1 -> Integrator/1
  Integrator/1 -> Add/2
  Gain/1 -> Add/1

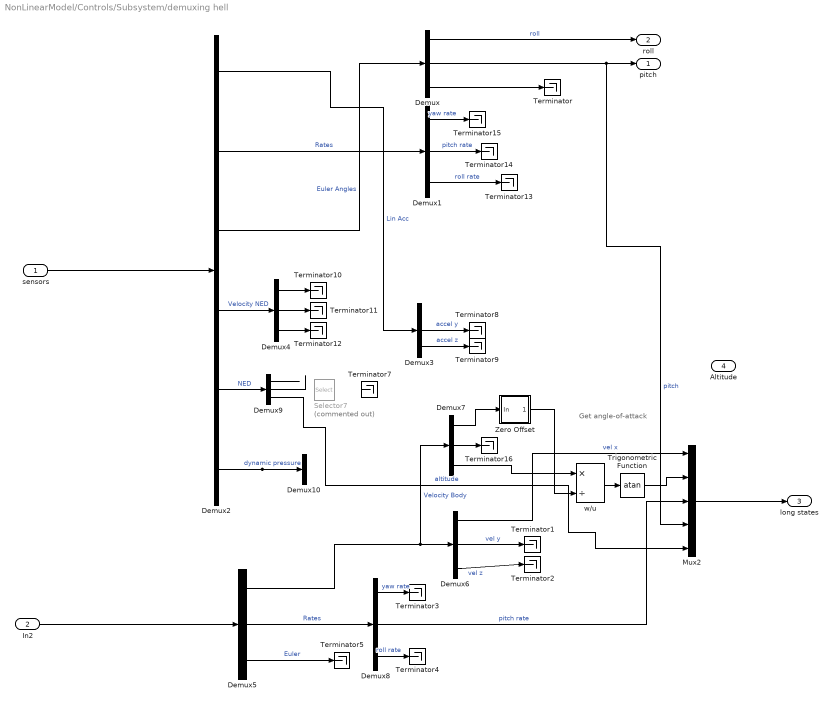
== system NonLinearModel/Controls/Subsystem/demuxing hell ==
  note: Get angle-of-attack
  sensors : Inport
  In2 : Inport  Port=2
  Demux{,1,3..9} (9 alike) : Demux  Outputs=3
      Demux7 settings: DisplayOption=none
  Demux10 : Demux  Outputs=1
  Demux2 : Demux  Outputs=6
  Mux2 : Mux  Inputs=5
  Selector7 : Selector  Commented=on  InputPortWidth=3  IndexOptions=Index vector (dialog)  Indices=3  OutputSizes=[(-2)]
  Terminator{,1..5,7..16} (16 alike) : Terminator
  Trigonometric Function : Trigonometry  Operator=atan
  Zero Offset : Subsystem  mask(Zero offset){tol=10^-6}
      mask prompts: tol "Tolerance"
      mask help: This block outputs a value equal to the tolerance specified in the block parameters if the input falls within a sphere with this tolerance as radius and center in the origin. Otherwise, the output equals the input.
      mask Help: This block outputs a value equal to the tolerance specified in the block parameters if the input falls within a sphere with this tolerance as radius and center in the origin. Otherwise, the output equals the input.
  w/u : Product  Inputs=*/  InputSameDT=on  SaturateOnIntegerOverflow=on  OutDataTypeStr=Inherit: Same as first input
  pitch : Outport
  roll : Outport  Port=2
  long states : Outport  Port=3
  Altitude : Outport  Port=4
  wires:
  Demux8/3 -> Terminator4/1  "roll rate"
  Demux5/1 -> Demux7/1, Demux6/1  "Velocity Body"
  Demux/3 -> Terminator/1
  Demux1/2 -> Terminator14/1  "pitch rate"
  Demux2/1 -> Demux3/1  "Lin Acc"
  Demux4/2 -> Terminator11/1
  w/u/1 -> Trigonometric Function/1
  Demux7/2 -> Terminator16/1
  Demux7/1 -> Zero Offset/1(In)
  Demux4/1 -> Terminator10/1
  Demux6/2 -> Terminator1/1  "vel y"
  Trigonometric Function/1 -> Mux2/2
  Demux2/5 -> Demux9/1  "NED"
  Demux2/2 -> Demux1/1  "Rates"
  Demux4/3 -> Terminator12/1
  Demux/2 -> Mux2/4, pitch/1  "pitch"
  Demux8/1 -> Terminator3/1  "yaw rate"
  Demux1/3 -> Terminator13/1  "roll rate"
  Demux5/2 -> Demux8/1  "Rates"
  Demux2/3 -> Demux/1  "Euler Angles"
  Demux3/3 -> Terminator9/1  "accel z"
  Demux2/4 -> Demux4/1  "Velocity NED"
  Demux3/2 -> Terminator8/1  "accel y"
  Demux8/2 -> Mux2/3  "pitch rate"
  Zero Offset/1(Out) -> w/u/2
  Demux7/3 -> w/u/1
  Mux2/1 -> long states/1
  Demux6/1 -> Mux2/1  "vel x"
  Demux6/3 -> Terminator2/1  "vel z"
  Demux5/3 -> Terminator5/1  "Euler"
  Demux2/6 -> Demux10/1  "dynamic pressure"
  Demux1/1 -> Terminator15/1  "yaw rate"
  Demux/1 -> roll/1  "roll"
  sensors/1 -> Demux2/1
  In2/1 -> Demux5/1
  Demux9/3 -> Mux2/5  "altitude"
  Demux9/1 -> ?
  Demux9/2 -> ?

== system NonLinearModel/My Aircraft/Aerodynamic model/Aerodynamic Force ==
  note: Get aerodynamic forces in
      | wind axes
  CD : Inport  PortDimensions=1
  CY : Inport  Port=2  PortDimensions=1
  CL : Inport  Port=3  PortDimensions=1
  pdyn : Inport  Port=4  PortDimensions=1
  ChSign : Gain  Gain=-1  SaturateOnIntegerOverflow=on  OutDataTypeStr=Inherit: Same as input  ParamDataTypeStr=Inherit: Same as input
  ChSign1 : Gain  Gain=-1  SaturateOnIntegerOverflow=on  OutDataTypeStr=Inherit: Same as input  ParamDataTypeStr=Inherit: Same as input
  Mux : Mux  Inputs=3
  Product : Product  Inputs=3  InputSameDT=on  SaturateOnIntegerOverflow=on  OutDataTypeStr=Inherit: Same as first input
  Wing area : Constant  Value=S
  Faero : Outport
  wires:
  Wing area/1 -> Product/3
  pdyn/1 -> Product/2
  Mux/1 -> Product/1
  CL/1 -> ChSign1/1
  CY/1 -> Mux/2
  CD/1 -> ChSign/1
  ChSign/1 -> Mux/1
  ChSign1/1 -> Mux/3
  Product/1 -> Faero/1

== system NonLinearModel/My Aircraft/Aerodynamic model/Aerodynamic Moment ==
  note: Output
  note: Compute moments
  note: Sources
  Cl : Inport  PortDimensions=1
  Cm : Inport  Port=2  PortDimensions=1
  Cn : Inport  Port=3  PortDimensions=1
  pdyn : Inport  Port=4  PortDimensions=1
  Mux : Mux  Inputs=3
  Pitch : Product  Inputs=4  InputSameDT=on  SaturateOnIntegerOverflow=on  OutDataTypeStr=Inherit: Same as first input
  Roll : Product  Inputs=4  InputSameDT=on  SaturateOnIntegerOverflow=on  OutDataTypeStr=Inherit: Same as first input
  Wing area : Constant  Value=S
  Wing chord : Constant  Value=c
  Wing span : Constant  Value=b
  Yaw : Product  Inputs=4  InputSameDT=on  SaturateOnIntegerOverflow=on  OutDataTypeStr=Inherit: Same as first input
  Maero : Outport
  wires:
  Yaw/1 -> Mux/3
  Pitch/1 -> Mux/2
  Mux/1 -> Maero/1
  Roll/1 -> Mux/1
  Wing span/1 -> Yaw/3, Roll/3
  Wing chord/1 -> Pitch/3
  Wing area/1 -> Yaw/2, Pitch/2, Roll/2
  pdyn/1 -> Yaw/1, Pitch/1, Roll/1
  Cn/1 -> Yaw/4
  Cm/1 -> Pitch/4
  Cl/1 -> Roll/4

== system NonLinearModel/My Aircraft/Aerodynamic model/Dynamic Pressure ==
  WindAxesVel : Inport  PortDimensions=[3 1]
  rho : Inport  Port=2  PortDimensions=1
  0.5*rho*Va^2 : Product  InputSameDT=on  SaturateOnIntegerOverflow=on  OutDataTypeStr=Inherit: Same as first input
  Demux : Demux  Outputs=3
      settings: DisplayOption=none
  Gain : Gain  Gain=1/2  SaturateOnIntegerOverflow=on  OutDataTypeStr=Inherit: Same as input  ParamDataTypeStr=Inherit: Same as input
  Terminator : Terminator
  Terminator1 : Terminator
  Va^2 : Math  Operator=square  SignedPower=on
  pdyn : Outport
  wires:
  0.5*rho*Va^2/1 -> pdyn/1
  Gain/1 -> 0.5*rho*Va^2/2
  Va^2/1 -> 0.5*rho*Va^2/1
  WindAxesVel/1 -> Demux/1
  Demux/2 -> Terminator/1
  Demux/3 -> Terminator1/1
  rho/1 -> Gain/1
  Demux/1 -> Va^2/1

== system NonLinearModel/My Aircraft/Aerodynamic model/Wind-axes Velocities ==
  note: Get angle-of-attack
  note: Sources
  Vbody : Inport  PortDimensions=[3 1]
  SoundSpd : Inport  Port=2  PortDimensions=1
  Demux : Demux  Outputs=3
      settings: DisplayOption=none
  Derivative : Derivative
  Mux : Mux  Inputs=3
  Mux1 : Mux  Inputs=2
  Trigonometric Function : Trigonometry  Operator=atan
  Trigonometric Function1 : Trigonometry  Operator=asin
  V/a : Product  Inputs=*/  InputSameDT=on  SaturateOnIntegerOverflow=on  OutDataTypeStr=Inherit: Same as first input
  Vector norm : Subsystem  mask(Vector norm-2){}
      mask help: Compute the 2-norm (magnitude) of a vector, |v| = sqrt(v'v).
      mask Help:
      | The block compute the 2-norm (or magnitude) of a vector.
      | <P><B>Input:</B> nx1 vector;</P>
      | <P><B>Output:</B> scalar magnitude.</P>
  Zero Offset : Subsystem  mask(Zero offset){tol=10^-6}
      mask prompts: tol "Tolerance"
      mask help: This block outputs a value equal to the tolerance specified in the block parameters if the input falls within a sphere with this tolerance as radius and center in the origin. Otherwise, the output equals the input.
      mask Help: This block outputs a value equal to the tolerance specified in the block parameters if the input falls within a sphere with this tolerance as radius and center in the origin. Otherwise, the output equals the input.
  v/Va : Product  Inputs=*/  InputSameDT=on  SaturateOnIntegerOverflow=on  OutDataTypeStr=Inherit: Same as first input
  w/u : Product  Inputs=*/  InputSameDT=on  SaturateOnIntegerOverflow=on  OutDataTypeStr=Inherit: Same as first input
  WindAxesVel : Outport
  AlphaBetaDot : Outport  Port=2
  Mach : Outport  Port=3
  wires:
  Zero Offset/1(Out) -> w/u/2
  Mux/1 -> WindAxesVel/1
  v/Va/1 -> Trigonometric Function1/1
  w/u/1 -> Trigonometric Function/1
  Demux/3 -> w/u/1
  Demux/2 -> v/Va/1
  Demux/1 -> Zero Offset/1(In)
  Vbody/1 -> Vector norm/1(Vec), Demux/1
  Mux1/1 -> Derivative/1
  Derivative/1 -> AlphaBetaDot/1
  SoundSpd/1 -> V/a/2
  V/a/1 -> Mach/1
  Trigonometric Function/1 -> Mux/3, Mux1/1
  Vector norm/1(Mag) -> V/a/1, v/Va/2, Mux/1
  Trigonometric Function1/1 -> Mux/2, Mux1/2

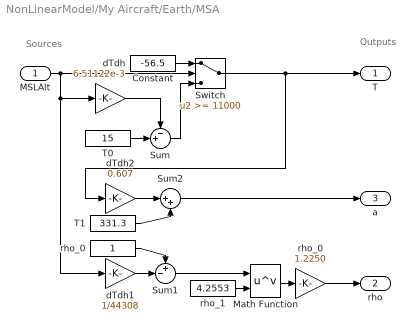
== system NonLinearModel/My Aircraft/Earth/MSA ==
  note: Sources
  note: Outputs
  MSLAlt : Inport  PortDimensions=1
  Constant : Constant  Value=-56.5
  Math Function : Math  Operator=pow  SignedPower=on
  Sum : Sum  Inputs=-+|
  Sum1 : Sum  Inputs=+-|
  Sum2 : Sum  Inputs=|++
  Switch : Switch  Threshold=11000  SaturateOnIntegerOverflow=off  InputSameDT=off
  T0 : Constant  Value=15
  T1 : Constant  Value=331.3
  dTdh : Gain  Gain=6.51122e-3
  dTdh1 : Gain  Gain=1/44308
  dTdh2 : Gain  Gain=0.607
  rho_0 : Constant
  "rho_0 " : Gain  Gain=1.2250
  rho_1 : Constant  Value=4.2553
  T : Outport
  rho : Outport  Port=2
  a : Outport  Port=3
  wires:
  Sum2/1 -> a/1
  T1/1 -> Sum2/2
  dTdh2/1 -> Sum2/1
  "rho_0 "/1 -> rho/1
  Math Function/1 -> "rho_0 "/1
  rho_1/1 -> Math Function/2
  Sum1/1 -> Math Function/1
  dTdh1/1 -> Sum1/2
  rho_0/1 -> Sum1/1
  Switch/1 -> dTdh2/1, T/1
  Sum/1 -> Switch/3
  dTdh/1 -> Sum/1
  T0/1 -> Sum/2
  Constant/1 -> Switch/1
  MSLAlt/1 -> dTdh1/1, dTdh/1, Switch/2

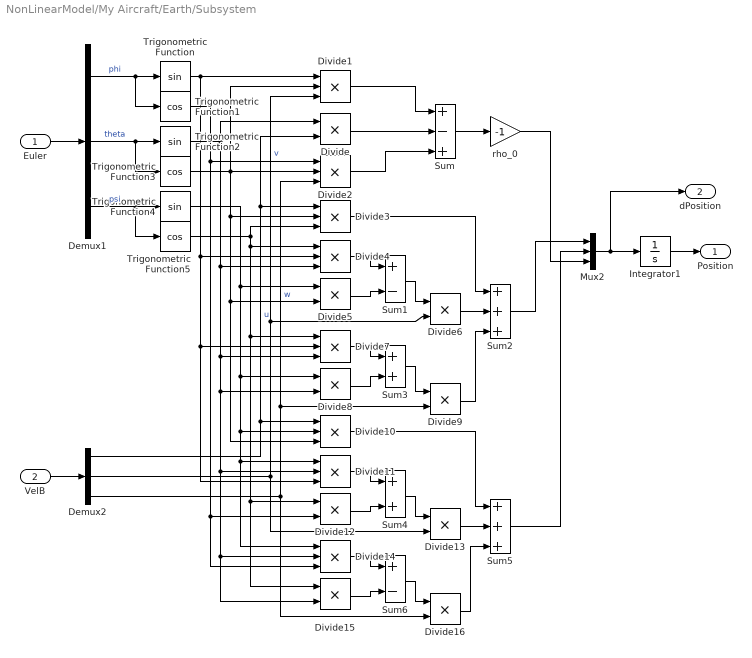
== system NonLinearModel/My Aircraft/Earth/Subsystem ==
  Euler : Inport
  VelB : Inport  Port=2
  Demux1 : Demux  Outputs=3
      settings: DisplayOption=none
  Demux2 : Demux  Outputs=3
      settings: DisplayOption=none
  Divide{,5..6,8..9,12..13,15..16} (9 alike) : Product  Inputs=**
  Divide{1..4,7,10..11,14} (8 alike) : Product  Inputs=3
  Integrator1 : Integrator  InitialCondition=[0 0 H_init]
  Mux2 : Mux  Inputs=3
  Sum : Sum  Inputs=+-+
  Sum1 : Sum  Inputs=+-
  Sum2 : Sum  Inputs=+++
  Sum3 : Sum
  Sum4 : Sum
  Sum5 : Sum  Inputs=+++
  Sum6 : Sum  Inputs=+-
  Trigonometric Function : Trigonometry
  Trigonometric Function1 : Trigonometry  Operator=cos
  Trigonometric Function2 : Trigonometry
  Trigonometric Function3 : Trigonometry  Operator=cos
  Trigonometric Function4 : Trigonometry
  Trigonometric Function5 : Trigonometry  Operator=cos
  "rho_0 " : Gain  Gain=-1
  Position : Outport
  dPosition : Outport  Port=2
  wires:
  Euler/1 -> Demux1/1
  VelB/1 -> Demux2/1
  Demux1/1 -> Trigonometric Function/1, Trigonometric Function1/1  "phi"
  Demux1/2 -> Trigonometric Function2/1, Trigonometric Function3/1  "theta"
  Demux1/3 -> Trigonometric Function4/1, Trigonometric Function5/1  "psi"
  Demux2/1 -> Divide/2, Divide3/1, Divide10/1  "u"
  Trigonometric Function2/1 -> Divide/1, Divide4/3, Divide7/3, Divide8/2, Divide11/2, Divide14/2, Divide15/2
  Trigonometric Function/1 -> Divide1/1, Divide4/2, Divide7/2, Divide11/3
  Demux2/2 -> Divide1/3, Divide6/2, Divide13/2  "v"
  Trigonometric Function3/1 -> Divide1/2, Divide2/2, Divide3/2, Divide5/2, Divide10/3
  Trigonometric Function1/1 -> Divide2/1, Divide12/2, Divide14/3
  Trigonometric Function4/1 -> Divide5/1, Divide8/1, Divide10/2, Divide11/1, Divide14/1
  Trigonometric Function5/1 -> Divide3/3, Divide4/1, Divide7/1, Divide12/1, Divide15/1
  Demux2/3 -> Divide2/3, Divide9/2, Divide16/2  "w"
  Divide1/1 -> Sum/1
  Divide/1 -> Sum/2
  Divide2/1 -> Sum/3
  Sum/1 -> "rho_0 "/1
  "rho_0 "/1 -> Mux2/3
  Divide3/1 -> Sum2/1
  Divide4/1 -> Sum1/1
  Divide5/1 -> Sum1/2
  Sum1/1 -> Divide6/1
  Divide6/1 -> Sum2/2
  Divide7/1 -> Sum3/1
  Divide8/1 -> Sum3/2
  Sum3/1 -> Divide9/1
  Divide9/1 -> Sum2/3
  Sum2/1 -> Mux2/1
  Divide10/1 -> Sum5/1
  Divide11/1 -> Sum4/1
  Divide12/1 -> Sum4/2
  Sum4/1 -> Divide13/1
  Divide13/1 -> Sum5/2
  Divide14/1 -> Sum6/1
  Divide15/1 -> Sum6/2
  Sum6/1 -> Divide16/1
  Divide16/1 -> Sum5/3
  Sum5/1 -> Mux2/2
  Mux2/1 -> Integrator1/1, dPosition/1
  Integrator1/1 -> Position/1

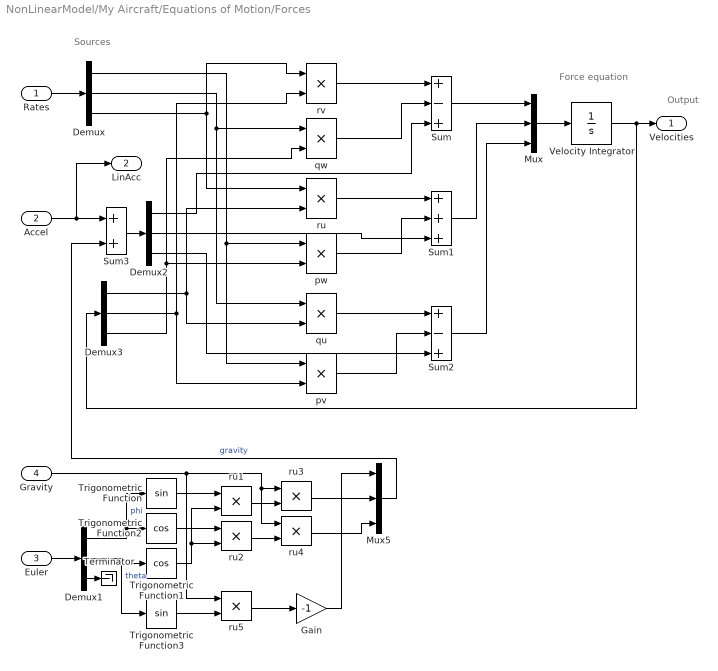
== system NonLinearModel/My Aircraft/Equations of Motion/Forces ==
  note: Sources
  note: Force equation
  note: Output
  Rates : Inport  PortDimensions=[3 1]
  Accel : Inport  Port=2  PortDimensions=[3 1]
  Euler : Inport  Port=3
  Gravity : Inport  Port=4  PortDimensions=1
  Demux{,1..3} (4 alike) : Demux  Outputs=3
      settings: DisplayOption=none
  Gain : Gain  Gain=-1
  Mux : Mux  Inputs=3
  Mux5 : Mux  Inputs=3
  Sum : Sum  Inputs=+-+  InputSameDT=on  SaturateOnIntegerOverflow=on  OutDataTypeStr=Inherit: Same as first input
  Sum1 : Sum  Inputs=+++  InputSameDT=on  SaturateOnIntegerOverflow=on  OutDataTypeStr=Inherit: Same as first input
  Sum2 : Sum  Inputs=+-+  InputSameDT=on  SaturateOnIntegerOverflow=on  OutDataTypeStr=Inherit: Same as first input
  Sum3 : Sum  InputSameDT=on  SaturateOnIntegerOverflow=on  OutDataTypeStr=Inherit: Same as first input
  Terminator : Terminator
  Trigonometric Function : Trigonometry
  Trigonometric Function1 : Trigonometry  Operator=cos
  Trigonometric Function2 : Trigonometry  Operator=cos
  Trigonometric Function3 : Trigonometry
  Velocity Integrator : Integrator  InitialCondition=VelocitiesIni
  pv : Product  InputSameDT=on  SaturateOnIntegerOverflow=on  OutDataTypeStr=Inherit: Same as first input
  pw : Product  InputSameDT=on  SaturateOnIntegerOverflow=on  OutDataTypeStr=Inherit: Same as first input
  qu : Product  InputSameDT=on  SaturateOnIntegerOverflow=on  OutDataTypeStr=Inherit: Same as first input
  qw : Product  InputSameDT=on  SaturateOnIntegerOverflow=on  OutDataTypeStr=Inherit: Same as first input
  ru{,1..5} (6 alike) : Product  InputSameDT=on  SaturateOnIntegerOverflow=on  OutDataTypeStr=Inherit: Same as first input
  rv : Product  InputSameDT=on  SaturateOnIntegerOverflow=on  OutDataTypeStr=Inherit: Same as first input
  Velocities : Outport
  LinAcc : Outport  Port=2
  wires:
  Sum3/1 -> Demux2/1
  qw/1 -> Sum/2
  rv/1 -> Sum/1
  Demux/1 -> pv/1, pw/1
  Demux/3 -> rv/1, ru/1
  Demux/2 -> qw/1, qu/1
  Rates/1 -> Demux/1
  Demux2/3 -> Sum2/3
  Demux2/2 -> Sum1/3
  ru/1 -> Sum1/1
  pw/1 -> Sum1/2
  qu/1 -> Sum2/1
  pv/1 -> Sum2/2
  Sum/1 -> Mux/1
  Sum1/1 -> Mux/2
  Sum2/1 -> Mux/3
  Mux/1 -> Velocity Integrator/1
  Demux3/1 -> qu/2, ru/2
  Demux3/2 -> pv/2, rv/2
  Demux3/3 -> qw/2, pw/2
  Euler/1 -> Demux1/1
  Demux1/3 -> Terminator/1
  Demux1/1 -> Trigonometric Function2/1, Trigonometric Function/1  "phi"
  Trigonometric Function2/1 -> ru2/1
  ru1/1 -> ru3/2
  ru2/1 -> ru4/2
  ru5/1 -> Gain/1
  Mux5/1 -> Sum3/2  "gravity"
  Gravity/1 -> ru5/1, ru3/1, ru4/1
  Gain/1 -> Mux5/1
  ru4/1 -> Mux5/3
  ru3/1 -> Mux5/2
  Trigonometric Function1/1 -> ru1/2, ru2/2
  Velocity Integrator/1 -> Velocities/1, Demux3/1
  Accel/1 -> Sum3/1, LinAcc/1
  Demux2/1 -> Sum/3
  Trigonometric Function3/1 -> ru5/2
  Demux1/2 -> Trigonometric Function1/1, Trigonometric Function3/1  "theta"
  Trigonometric Function/1 -> ru1/1

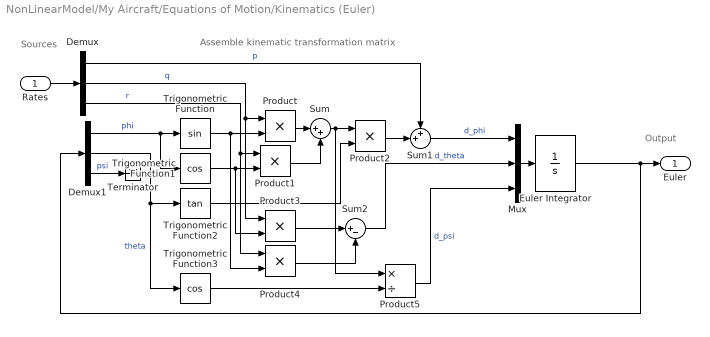
== system NonLinearModel/My Aircraft/Equations of Motion/Kinematics (Euler) ==
  note: Output
  note: Sources
  note: Assemble kinematic transformation matrix
  Rates : Inport
  Demux : Demux  Outputs=3
      settings: DisplayOption=none
  Demux1 : Demux  Outputs=3
      settings: DisplayOption=none
  Euler Integrator : Integrator  InitialCondition=EulerIniX'
  Mux : Mux  Inputs=3
  Product{,1..4} (5 alike) : Product  RndMeth=Zero
  Product5 : Product  Inputs=*/  RndMeth=Zero
  Sum : Sum  Inputs=|++
  Sum1 : Sum  Inputs=++|
  Sum2 : Sum  Inputs=|+-
  Terminator : Terminator
  Trigonometric Function : Trigonometry
  Trigonometric Function1 : Trigonometry  Operator=cos
  Trigonometric Function2 : Trigonometry  Operator=tan
  Trigonometric Function3 : Trigonometry  Operator=cos
  Euler : Outport
  wires:
  Rates/1 -> Demux/1
  Demux/1 -> Sum1/1  "p"
  Demux/3 -> Product1/1, Product4/1  "r"
  Demux1/1 -> Trigonometric Function/1, Trigonometric Function1/1  "phi"
  Demux1/2 -> Trigonometric Function2/1, Trigonometric Function3/1  "theta"
  Demux1/3 -> Terminator/1  "psi"
  Trigonometric Function/1 -> Product/2, Product4/2
  Trigonometric Function1/1 -> Product1/2, Product3/2
  Product/1 -> Sum/1
  Product1/1 -> Sum/2
  Sum/1 -> Product2/1, Product5/1
  Trigonometric Function2/1 -> Product2/2
  Product2/1 -> Sum1/2
  Product3/1 -> Sum2/1
  Product4/1 -> Sum2/2
  Mux/1 -> Euler Integrator/1
  Sum1/1 -> Mux/1  "d_phi"
  Sum2/1 -> Mux/2  "d_theta"
  Trigonometric Function3/1 -> Product5/2
  Product5/1 -> Mux/3  "d_psi"
  Demux/2 -> Product/1, Product3/1  "q"
  Euler Integrator/1 -> Demux1/1, Euler/1
